simulink model "lab7_t18"  (R2021a)
settings: Solver=VariableStepAuto  StartTime=0.0  StopTime=10.0  RelTol=1e-3
libraries: simulink x1
settings Model: Creator=reemb  LastModifiedBy=reemb

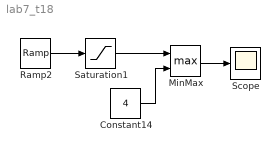
== system lab7_t18 ==
  Constant14 : Constant  Value=4
  MinMax : MinMax  Function=max  Inputs=2
  Ramp2 : simulink/Sources/Ramp  slope=2  start=0  InitialOutput=0
  Saturation1 : Saturate  UpperLimit=10  LowerLimit=0
  Scope : Scope
  wires:
  MinMax/1 -> Scope/1
  Ramp2/1 -> Saturation1/1
  Constant14/1 -> MinMax/2
  Saturation1/1 -> MinMax/1
